simulink model "galvo_model_test"  (R2021a)
settings: Solver=VariableStepAuto  StartTime=0.0  StopTime=20  RelTol=1e-3
settings Model: Creator=billy  LastModifiedBy=billy

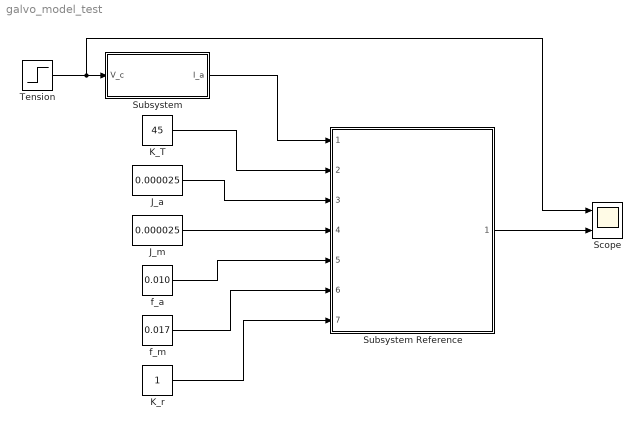
== system galvo_model_test ==
  J_a : Constant  Value=0.000025
  J_m : Constant  Value=0.000025
  K_T : Constant  Value=45  LockScale=on
  K_r : Constant
  Scope : Scope  NumInputPorts=2
  Subsystem : Subsystem
  Subsystem Reference : Subsystem  ReferencedSubsystem=galvo_cao
  Tension : Step  After=0.125  SampleTime=0
  f_a : Constant  Value=0.010
  f_m : Constant  Value=0.017
  wires:
  K_T/1 -> Subsystem Reference/2
  J_a/1 -> Subsystem Reference/3
  J_m/1 -> Subsystem Reference/4
  f_a/1 -> Subsystem Reference/5
  f_m/1 -> Subsystem Reference/6
  K_r/1 -> Subsystem Reference/7
  Subsystem/1(I_a) -> Subsystem Reference/1
  Subsystem Reference/1 -> Scope/2
  Tension/1 -> Scope/1, Subsystem/1(V_c)

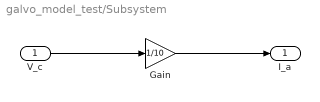
== system galvo_model_test/Subsystem ==
  V_c : Inport
  Gain : Gain  Gain=1/10
  I_a : Outport
  wires:
  V_c/1 -> Gain/1
  Gain/1 -> I_a/1
